simulink model "dcmotor_speed"  (R2019a)
settings: Solver=VariableStepAuto  StartTime=0.0  StopTime=2  RelTol=1e-5
values from neighbouring files (symbols this model uses):
  b = 0.1    [dcmotor_speed.m]    (also in dcmotorspeed_pid.m)
  J = 0.01    [dcmotor_speed.m]    (also in dcmotorspeed_pid.m)
  K = 0.01    [dcmotor_speed.m]    (also in dcmotorspeed_pid.m)
  L = 0.5    [dcmotor_speed.m]    (also in dcmotorspeed_pid.m)
  R = 1    [dcmotor_speed.m]    (also in dcmotorspeed_pid.m)
settings Model: Creator=dağlar  LastModifiedBy=dağlar

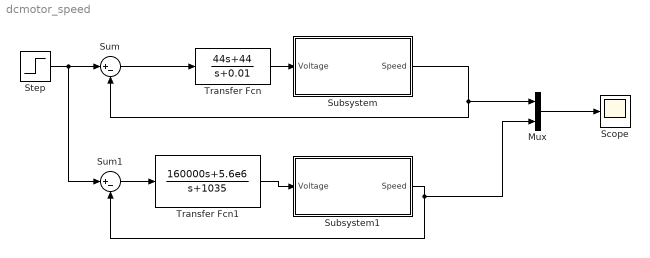
== system dcmotor_speed ==
  Mux : Mux  Inputs=2
  Scope : Scope
  Step : Step  Time=0  SampleTime=0
  Subsystem : Subsystem
  Subsystem1 : Subsystem
  Sum : Sum  Inputs=|+-
  Sum1 : Sum  Inputs=|+-
  Transfer Fcn : TransferFcn  Numerator=[44 44]  Denominator=[1 0.01]
  Transfer Fcn1 : TransferFcn  Numerator=[160000 5.6e6]  Denominator=[1 1035]
  wires:
  Subsystem/1(Speed) -> Mux/1, Sum/2
  Step/1 -> Sum1/1, Sum/1
  Sum/1 -> Transfer Fcn/1
  Transfer Fcn/1 -> Subsystem/1("Voltage ")
  Transfer Fcn1/1 -> Subsystem1/1("Voltage ")
  Sum1/1 -> Transfer Fcn1/1
  Subsystem1/1(Speed) -> Mux/2, Sum1/2
  Mux/1 -> Scope/1

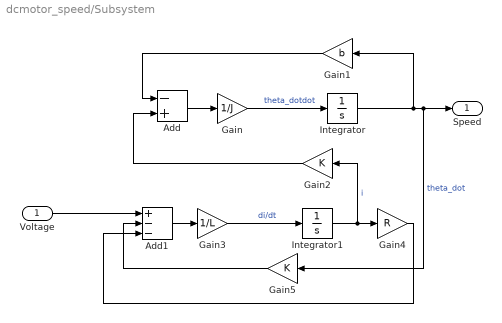
== system dcmotor_speed/Subsystem ==
  "Voltage " : Inport
  Add : Sum  Inputs=-+
  Add1 : Sum  Inputs=+--
  Gain : Gain  Gain=1/J
  Gain1 : Gain  Gain=b
  Gain2 : Gain  Gain=K
  Gain3 : Gain  Gain=1/L
  Gain4 : Gain  Gain=R
  Gain5 : Gain  Gain=K
  Integrator : Integrator
  Integrator1 : Integrator
  Speed : Outport
  wires:
  "Voltage "/1 -> Add1/1
  Gain2/1 -> Add/2
  Integrator1/1 -> Gain4/1, Gain2/1  "i"
  Add1/1 -> Gain3/1
  Gain4/1 -> Add1/3
  Gain/1 -> Integrator/1  "theta_dotdot"
  Gain5/1 -> Add1/2
  Add/1 -> Gain/1
  Integrator/1 -> Speed/1, Gain5/1, Gain1/1  "theta_dot"
  Gain1/1 -> Add/1
  Gain3/1 -> Integrator1/1  "di/dt"

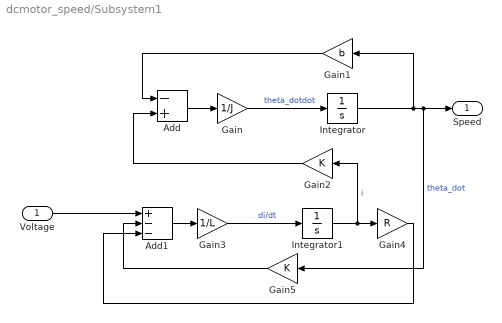
== system dcmotor_speed/Subsystem1 ==
  "Voltage " : Inport
  Add : Sum  Inputs=-+
  Add1 : Sum  Inputs=+--
  Gain : Gain  Gain=1/J
  Gain1 : Gain  Gain=b
  Gain2 : Gain  Gain=K
  Gain3 : Gain  Gain=1/L
  Gain4 : Gain  Gain=R
  Gain5 : Gain  Gain=K
  Integrator : Integrator
  Integrator1 : Integrator
  Speed : Outport
  wires:
  "Voltage "/1 -> Add1/1
  Gain2/1 -> Add/2
  Integrator1/1 -> Gain4/1, Gain2/1  "i"
  Add1/1 -> Gain3/1
  Gain4/1 -> Add1/3
  Gain/1 -> Integrator/1  "theta_dotdot"
  Gain5/1 -> Add1/2
  Add/1 -> Gain/1
  Integrator/1 -> Speed/1, Gain5/1, Gain1/1  "theta_dot"
  Gain1/1 -> Add/1
  Gain3/1 -> Integrator1/1  "di/dt"
